simulink model "control_system"  (R2020b)
settings: Solver=FixedStepAuto  StartTime=0.0  StopTime=t_sim  FixedStep=Ts  RelTol=1e-2
values from neighbouring files (symbols this model uses):
  Hp = 10    [main_script.m]
  InitPosX = -2.4980e+03    (= -2498)    [main_script.m]
  InitPosY = -650.5503    [main_script.m]
  InitVelX = V0*cosd(InitYaw)    [main_script.m]
  InitVelY = V0*sind(InitYaw)    [main_script.m]
  InitYaw = 21    [main_script.m]
  lr = 1.592    [main_script.m]
  m = 1625    [main_script.m]
  Ts = 0.1    [main_script.m]
  V0 = 25    [main_script.m]
libraries: neural x856, simulink x1, autolibshared x1, drivingscenarioandsensors x1
(part 6 of 40)

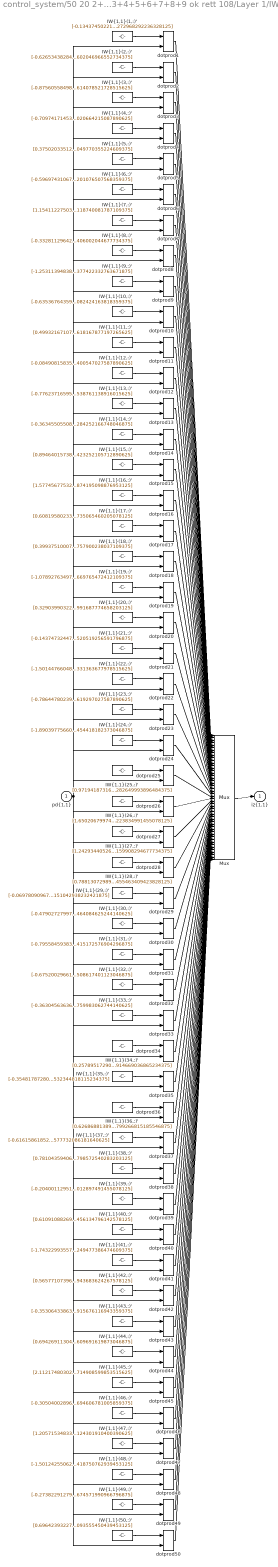
== system control_system/50 20 2+3+4+5+6+7+8+9 ok rett 108/Layer 1/IW{1,1} ==
  "pd{1,1}" : Inport  PortDimensions=9  SampleTime=0.1
      mask Display: e = 0.06;c1 = [120 230 180]/255;c2 = ([120 230 180]+0)/(256+128);c3 = ([120 230 180]+128)/(256+128);patch([0 1 1 0],[0 0 1 1],c1);patch([0 1 1 1-e 1-e 0+e],[0 0 1 1-e 0+e 0+e],c2);patch([0 0 1 1-e 0+e 0+e],[0 1 1 1-e 1-e 0+e],c3);plot([0 1 1 0 0],[0 0 1 1 0]);
  "IW{1,1}(1,:)'" : Constant  Value=[-0.1343745022107840358938091185336816124618053436279296875;-0.2201570215463205248962452742489404045045375823974609375;0.493314924472624927176411802065558731555938720703125;0.240218537769716855567736502052866853773593902587890625;0.0035729013340322856272235352292909738025628030300140380859375;1.2275952974377080106904713829862885177135467529296875;0.32609691089661685392542267436510883271694183349609375;-0.9495712296454932310751928525860421359539031982421875;-0.70107606410829692578090543975122272968292236328125]
      mask Display: e = 0.06;c1 = [120 150 230]/255;c2 = ([120 150 230]+0)/383;c3 = ([120 150 230]+128)/383;patch([0 1 1 0],[0 0 1 1],c1);patch([0 1 1 1-e 1-e 0+e],[0 0 1 1-e 0+e 0+e],c2);patch([0 0 1 1-e 0+e 0+e],[0 1 1 1-e 1-e 0+e],c3);plot([0 1 1 0 0],[0 0 1 1 0]);disp('Weights');
  "IW{1,1}(10,:)'" : Constant  Value=[-0.635367643598796494330827044905163347721099853515625;1.266134724639150999081493864650838077068328857421875;0.279110981570210359148376255689072422683238983154296875;0.6725165935042671794263924311962909996509552001953125;-0.279299335778829205256812429070123471319675445556640625;0.1298072467704776411512312961349380202591419219970703125;0.79908196252433827400096788551309145987033843994140625;1.35790638049596434910881725954823195934295654296875;0.0948926349490134268815921814166358672082424163818359375]
      mask Display: e = 0.06;c1 = [120 150 230]/255;c2 = ([120 150 230]+0)/383;c3 = ([120 150 230]+128)/383;patch([0 1 1 0],[0 0 1 1],c1);patch([0 1 1 1-e 1-e 0+e],[0 0 1 1-e 0+e 0+e],c2);patch([0 0 1 1-e 0+e 0+e],[0 1 1 1-e 1-e 0+e],c3);plot([0 1 1 0 0],[0 0 1 1 0]);disp('Weights');
  "IW{1,1}(11,:)'" : Constant  Value=[0.4993216710750658648976241238415241241455078125;0.5262356768534541817672334218514151871204376220703125;0.681666886525891246861874606111086905002593994140625;-0.87555884751066026527865915340953506529331207275390625;-0.60105755257610093966746944715850986540317535400390625;0.5843485194005146876605749639566056430339813232421875;0.96478303636410756016772438670159317553043365478515625;0.77348642815128221261744556613848544657230377197265625;-0.6497149588995887459219602533266879618167877197265625]
      mask Display: e = 0.06;c1 = [120 150 230]/255;c2 = ([120 150 230]+0)/383;c3 = ([120 150 230]+128)/383;patch([0 1 1 0],[0 0 1 1],c1);patch([0 1 1 1-e 1-e 0+e],[0 0 1 1-e 0+e 0+e],c2);patch([0 0 1 1-e 0+e 0+e],[0 1 1 1-e 1-e 0+e],c3);plot([0 1 1 0 0],[0 0 1 1 0]);disp('Weights');
  "IW{1,1}(12,:)'" : Constant  Value=[-0.084908158355977925157986874182824976742267608642578125;-0.7864413820746027905528308110660873353481292724609375;-1.011454847098846254738191419164650142192840576171875;-0.1117623118762176848139944240756449289619922637939453125;-0.207538480609310960200986073687090538442134857177734375;1.05662315566693099100348263164050877094268798828125;-1.27361323393598535602677657152526080608367919921875;-0.94238788342574653089656067095347680151462554931640625;-0.0740762271510614633829305830658995546400547027587890625]
      mask Display: e = 0.06;c1 = [120 150 230]/255;c2 = ([120 150 230]+0)/383;c3 = ([120 150 230]+128)/383;patch([0 1 1 0],[0 0 1 1],c1);patch([0 1 1 1-e 1-e 0+e],[0 0 1 1-e 0+e 0+e],c2);patch([0 0 1 1-e 0+e 0+e],[0 1 1 1-e 1-e 0+e],c3);plot([0 1 1 0 0],[0 0 1 1 0]);disp('Weights');
  "IW{1,1}(13,:)'" : Constant  Value=[-0.77623716595878800017516141451778821647167205810546875;0.01224940877890513639403291534790696459822356700897216796875;-1.1967390742769350442387121802312321960926055908203125;0.674325482748454163584028719924390316009521484375;-0.31108072366164207789296369810472242534160614013671875;-0.6359597085702881624769133850350044667720794677734375;-1.128846677766122130748271956690587103366851806640625;-0.006871567558858683588685067888945923186838626861572265625;-0.264283133847268258964646747699589468538761138916015625]
      mask Display: e = 0.06;c1 = [120 150 230]/255;c2 = ([120 150 230]+0)/383;c3 = ([120 150 230]+128)/383;patch([0 1 1 0],[0 0 1 1],c1);patch([0 1 1 1-e 1-e 0+e],[0 0 1 1-e 0+e 0+e],c2);patch([0 0 1 1-e 0+e 0+e],[0 1 1 1-e 1-e 0+e],c3);plot([0 1 1 0 0],[0 0 1 1 0]);disp('Weights');
  "IW{1,1}(14,:)'" : Constant  Value=[-0.363455055082136324617891887100995518267154693603515625;1.286478296564485201969318950432352721691131591796875;0.040608931980886768531302521978432196192443370819091796875;-0.304597316839120890730185919892392121255397796630859375;0.189441761685817888771765638011856935918331146240234375;-0.11649603633906462085700894704132224433124065399169921875;1.216577309348745306039063507341779768466949462890625;-2.649690499494823381354535740683786571025848388671875;-1.0884535716017775808239775869878940284252166748046875]
      mask Display: e = 0.06;c1 = [120 150 230]/255;c2 = ([120 150 230]+0)/383;c3 = ([120 150 230]+128)/383;patch([0 1 1 0],[0 0 1 1],c1);patch([0 1 1 1-e 1-e 0+e],[0 0 1 1-e 0+e 0+e],c2);patch([0 0 1 1-e 0+e 0+e],[0 1 1 1-e 1-e 0+e],c3);plot([0 1 1 0 0],[0 0 1 1 0]);disp('Weights');
  "IW{1,1}(15,:)'" : Constant  Value=[0.89464015738325664006680426609818823635578155517578125;0.81871186647511307032942795558483339846134185791015625;0.034969645491070143472622788749504252336919307708740234375;0.813319109544075491413650524918921291828155517578125;0.304501924088689202019253343678428791463375091552734375;1.276721925975607074832396392594091594219207763671875;0.376418920830022762924471635415102355182170867919921875;0.20670604322129293439758157546748407185077667236328125;1.1612427578136479411341497325338423252105712890625]
      mask Display: e = 0.06;c1 = [120 150 230]/255;c2 = ([120 150 230]+0)/383;c3 = ([120 150 230]+128)/383;patch([0 1 1 0],[0 0 1 1],c1);patch([0 1 1 1-e 1-e 0+e],[0 0 1 1-e 0+e 0+e],c2);patch([0 0 1 1-e 0+e 0+e],[0 1 1 1-e 1-e 0+e],c3);plot([0 1 1 0 0],[0 0 1 1 0]);disp('Weights');
  "IW{1,1}(16,:)'" : Constant  Value=[1.57745677532034367374080829904414713382720947265625;-1.1514762186593205939288964145816862583160400390625;0.9935027681728108017722433942253701388835906982421875;0.8910553917919352695520274210139177739620208740234375;0.474810013596444091543702370472601614892482757568359375;0.8601933682805522618508575760642997920513153076171875;0.332891623686451365582428252309910021722316741943359375;1.2544283751669607074319401363027282059192657470703125;-0.300158428375610075722335068348911590874195098876953125]
      mask Display: e = 0.06;c1 = [120 150 230]/255;c2 = ([120 150 230]+0)/383;c3 = ([120 150 230]+128)/383;patch([0 1 1 0],[0 0 1 1],c1);patch([0 1 1 1-e 1-e 0+e],[0 0 1 1-e 0+e 0+e],c2);patch([0 0 1 1-e 0+e 0+e],[0 1 1 1-e 1-e 0+e],c3);plot([0 1 1 0 0],[0 0 1 1 0]);disp('Weights');
  "IW{1,1}(17,:)'" : Constant  Value=[0.608195802333024726493704292806796729564666748046875;0.47127526029324162681888310544309206306934356689453125;0.36214244417380092588842899203882552683353424072265625;0.3294693882679109453448518252116627991199493408203125;-0.66612419048444915237183749923133291304111480712890625;0.5817769197731477159862834014347754418849945068359375;1.5236633537899508805679715806036256253719329833984375;-0.91766798575549302086074021644890308380126953125;0.88163371330469708642141313248430378735065460205078125]
      mask Display: e = 0.06;c1 = [120 150 230]/255;c2 = ([120 150 230]+0)/383;c3 = ([120 150 230]+128)/383;patch([0 1 1 0],[0 0 1 1],c1);patch([0 1 1 1-e 1-e 0+e],[0 0 1 1-e 0+e 0+e],c2);patch([0 0 1 1-e 0+e 0+e],[0 1 1 1-e 1-e 0+e],c3);plot([0 1 1 0 0],[0 0 1 1 0]);disp('Weights');
  "IW{1,1}(18,:)'" : Constant  Value=[0.399375100074075894962533084253664128482341766357421875;1.3435825717445688542994730596547015011310577392578125;1.5781318163517810138074537462671287357807159423828125;-0.155094863392196469220607468741945922374725341796875;1.3897167318388150558661209288402460515499114990234375;0.66382684499126110022615421257796697318553924560546875;-0.1403045882415885625693618976583820767700672149658203125;0.633292869042725303785346113727428019046783447265625;-1.19177375240624083829743540263734757900238037109375]
      mask Display: e = 0.06;c1 = [120 150 230]/255;c2 = ([120 150 230]+0)/383;c3 = ([120 150 230]+128)/383;patch([0 1 1 0],[0 0 1 1],c1);patch([0 1 1 1-e 1-e 0+e],[0 0 1 1-e 0+e 0+e],c2);patch([0 0 1 1-e 0+e 0+e],[0 1 1 1-e 1-e 0+e],c3);plot([0 1 1 0 0],[0 0 1 1 0]);disp('Weights');
  "IW{1,1}(19,:)'" : Constant  Value=[-1.0789276349723007086822690325789153575897216796875;-1.3867166392141216935129932608106173574924468994140625;0.1648811111358275127702910367588629014790058135986328125;-1.5050692494481001659778485191054642200469970703125;-0.403242892039837930173717950310674495995044708251953125;-0.0850366986317305506570818351974594406783580780029296875;0.351782679257654662396959110992611385881900787353515625;1.85432216169652708259718565386720001697540283203125;-0.399103180886815456229754772721207700669765472412109375]
      mask Display: e = 0.06;c1 = [120 150 230]/255;c2 = ([120 150 230]+0)/383;c3 = ([120 150 230]+128)/383;patch([0 1 1 0],[0 0 1 1],c1);patch([0 1 1 1-e 1-e 0+e],[0 0 1 1-e 0+e 0+e],c2);patch([0 0 1 1-e 0+e 0+e],[0 1 1 1-e 1-e 0+e],c3);plot([0 1 1 0 0],[0 0 1 1 0]);disp('Weights');
  "IW{1,1}(2,:)'" : Constant  Value=[-0.6265343828480018917304050773964263498783111572265625;-0.098149421145493020990357990740449167788028717041015625;1.9729387189784401979153471984318457543849945068359375;1.3105035919609397954133100938634015619754791259765625;-0.300689271275498715141338834655471146106719970703125;0.54673346645999842952079461610992439091205596923828125;-1.00482267753112264330184189020656049251556396484375;0.005126759769235396564657225582095634308643639087677001953125;0.402468829493407065367449604309513233602046966552734375]
      mask Display: e = 0.06;c1 = [120 150 230]/255;c2 = ([120 150 230]+0)/383;c3 = ([120 150 230]+128)/383;patch([0 1 1 0],[0 0 1 1],c1);patch([0 1 1 1-e 1-e 0+e],[0 0 1 1-e 0+e 0+e],c2);patch([0 0 1 1-e 0+e 0+e],[0 1 1 1-e 1-e 0+e],c3);plot([0 1 1 0 0],[0 0 1 1 0]);disp('Weights');
  "IW{1,1}(20,:)'" : Constant  Value=[0.32903990322955412040073497337289154529571533203125;0.58040702305057123577824995663831941783428192138671875;-1.079543369998765545147989541874267160892486572265625;0.495549709433944496339563556830398738384246826171875;0.01475849541834454471678217402086374931968748569488525390625;0.6517370707739134072511433259933255612850189208984375;0.7060091982681002686916826860397122800350189208984375;0.10264173611011488673749880717878113500773906707763671875;-1.34879506457316011847069603390991687774658203125]
      mask Display: e = 0.06;c1 = [120 150 230]/255;c2 = ([120 150 230]+0)/383;c3 = ([120 150 230]+128)/383;patch([0 1 1 0],[0 0 1 1],c1);patch([0 1 1 1-e 1-e 0+e],[0 0 1 1-e 0+e 0+e],c2);patch([0 0 1 1-e 0+e 0+e],[0 1 1 1-e 1-e 0+e],c3);plot([0 1 1 0 0],[0 0 1 1 0]);disp('Weights');
  "IW{1,1}(21,:)'" : Constant  Value=[-0.14374732447989624350981330280774272978305816650390625;-0.0402954239318593920859967738579143770039081573486328125;0.38731319765238569896581566354143433272838592529296875;1.989037631719348997449969829176552593708038330078125;0.76381127679371407790398507131612859666347503662109375;0.71549694533983487776396259505418129265308380126953125;-1.3060389462663597459624043040093965828418731689453125;-0.700024507199966450343708856962621212005615234375;-0.2408662673477610371985946358108776621520519256591796875]
      mask Display: e = 0.06;c1 = [120 150 230]/255;c2 = ([120 150 230]+0)/383;c3 = ([120 150 230]+128)/383;patch([0 1 1 0],[0 0 1 1],c1);patch([0 1 1 1-e 1-e 0+e],[0 0 1 1-e 0+e 0+e],c2);patch([0 0 1 1-e 0+e 0+e],[0 1 1 1-e 1-e 0+e],c3);plot([0 1 1 0 0],[0 0 1 1 0]);disp('Weights');
  "IW{1,1}(22,:)'" : Constant  Value=[-1.5014476604894049227567620619083754718303680419921875;-0.412754505781206815218098427067161537706851959228515625;0.76830306281267202184181996926781721413135528564453125;0.70981824529789394606638097684481181204319000244140625;-0.393729968921678608051450964921968989074230194091796875;-0.1718600999554333041974274465246708132326602935791015625;-1.9073931269723607417887478732154704630374908447265625;2.973563560321208054659791741869412362575531005859375;-0.250064300015983731473312445814372040331363677978515625]
      mask Display: e = 0.06;c1 = [120 150 230]/255;c2 = ([120 150 230]+0)/383;c3 = ([120 150 230]+128)/383;patch([0 1 1 0],[0 0 1 1],c1);patch([0 1 1 1-e 1-e 0+e],[0 0 1 1-e 0+e 0+e],c2);patch([0 0 1 1-e 0+e 0+e],[0 1 1 1-e 1-e 0+e],c3);plot([0 1 1 0 0],[0 0 1 1 0]);disp('Weights');
  "IW{1,1}(23,:)'" : Constant  Value=[-0.78644780239899658713653707309276796877384185791015625;0.2039698093212249652150802603500778786838054656982421875;-0.535590127558683182229515296057797968387603759765625;0.53857933595635765211540046948357485234737396240234375;1.3515952770876420441226173352333717048168182373046875;-2.42589564569713633801484320429153740406036376953125;-0.17670141464765565242345246588229201734066009521484375;0.044122307358018086897999410211923532187938690185546875;-1.1806380640758258326883378686034120619297027587890625]
      mask Display: e = 0.06;c1 = [120 150 230]/255;c2 = ([120 150 230]+0)/383;c3 = ([120 150 230]+128)/383;patch([0 1 1 0],[0 0 1 1],c1);patch([0 1 1 1-e 1-e 0+e],[0 0 1 1-e 0+e 0+e],c2);patch([0 0 1 1-e 0+e 0+e],[0 1 1 1-e 1-e 0+e],c3);plot([0 1 1 0 0],[0 0 1 1 0]);disp('Weights');
  "IW{1,1}(24,:)'" : Constant  Value=[-1.8903977566011811450863433492486365139484405517578125;-0.1716829364750723507793139788191183470189571380615234375;0.19568944686699929480511173096601851284503936767578125;-0.92695327627895751643194444113760255277156829833984375;-0.94439922472159576471995023894123733043670654296875;4.158514021467741628157455124892294406890869140625;-0.59169238273870117250652356233331374824047088623046875;3.865002745752950108482082214322872459888458251953125;-0.486221855689500326302976418446633033454418182373046875]
      mask Display: e = 0.06;c1 = [120 150 230]/255;c2 = ([120 150 230]+0)/383;c3 = ([120 150 230]+128)/383;patch([0 1 1 0],[0 0 1 1],c1);patch([0 1 1 1-e 1-e 0+e],[0 0 1 1-e 0+e 0+e],c2);patch([0 0 1 1-e 0+e 0+e],[0 1 1 1-e 1-e 0+e],c3);plot([0 1 1 0 0],[0 0 1 1 0]);disp('Weights');
  "IW{1,1}(25,:)'" : Constant  Value=[0.97194187316870339632401964991004206240177154541015625;0.33655565599595582693126516460324637591838836669921875;-0.732350146859455986003695215913467109203338623046875;-0.5342568270652463535697052066097967326641082763671875;0.294284086829917745919971139301196672022342681884765625;-0.380858389058827351281166784247034229338169097900390625;0.90022726195886804134715930558741092681884765625;0.388889458274653154745692518190480768680572509765625;-0.7233772643939886393127380870282649993896484375]
      mask Display: e = 0.06;c1 = [120 150 230]/255;c2 = ([120 150 230]+0)/383;c3 = ([120 150 230]+128)/383;patch([0 1 1 0],[0 0 1 1],c1);patch([0 1 1 1-e 1-e 0+e],[0 0 1 1-e 0+e 0+e],c2);patch([0 0 1 1-e 0+e 0+e],[0 1 1 1-e 1-e 0+e],c3);plot([0 1 1 0 0],[0 0 1 1 0]);disp('Weights');
  "IW{1,1}(26,:)'" : Constant  Value=[1.650206799742701679889478327822871506214141845703125;0.2751440287276978313713016177644021809101104736328125;-0.08839072554119496716307224914999096654355525970458984375;1.8091355921185316990573710427270270884037017822265625;0.88793122285300063456503494307980872690677642822265625;2.161317142218055042945934474118985235691070556640625;0.062490739860500597868675498602897278033196926116943359375;-0.728816435986441302219418503227643668651580810546875;-0.441417895919521463543588879474555142223834991455078125]
      mask Display: e = 0.06;c1 = [120 150 230]/255;c2 = ([120 150 230]+0)/383;c3 = ([120 150 230]+128)/383;patch([0 1 1 0],[0 0 1 1],c1);patch([0 1 1 1-e 1-e 0+e],[0 0 1 1-e 0+e 0+e],c2);patch([0 0 1 1-e 0+e 0+e],[0 1 1 1-e 1-e 0+e],c3);plot([0 1 1 0 0],[0 0 1 1 0]);disp('Weights');
  "IW{1,1}(27,:)'" : Constant  Value=[1.2429344052620334704073457032791338860988616943359375;0.643092034237877197000443629804067313671112060546875;-0.02543692723731975913192826510567101649940013885498046875;2.35271190603658642004347711917944252490997314453125;-0.045149049836735226370887374969242955558001995086669921875;0.51151019332570635267387615385814569890499114990234375;-0.2492781695850741774389547344981110654771327972412109375;2.47668571726079989048230345360934734344482421875;0.332171884911200032686195982023491524159908294677734375]
      mask Display: e = 0.06;c1 = [120 150 230]/255;c2 = ([120 150 230]+0)/383;c3 = ([120 150 230]+128)/383;patch([0 1 1 0],[0 0 1 1],c1);patch([0 1 1 1-e 1-e 0+e],[0 0 1 1-e 0+e 0+e],c2);patch([0 0 1 1-e 0+e 0+e],[0 1 1 1-e 1-e 0+e],c3);plot([0 1 1 0 0],[0 0 1 1 0]);disp('Weights');
  "IW{1,1}(28,:)'" : Constant  Value=[0.788130729896838300163608437287621200084686279296875;-0.2054429587058503869911874062381684780120849609375;-0.4717687480737471350522582724806852638721466064453125;-0.5514851259956536910777913362835533916950225830078125;1.2579968231444536019836277773720212280750274658203125;3.53449811365294674914139250176958739757537841796875;-0.05000756981324182282033774527008063159883022308349609375;1.066653902632202832734265030012466013431549072265625;-0.92112634419193384349711095637758262455463409423828125]
      mask Display: e = 0.06;c1 = [120 150 230]/255;c2 = ([120 150 230]+0)/383;c3 = ([120 150 230]+128)/383;patch([0 1 1 0],[0 0 1 1],c1);patch([0 1 1 1-e 1-e 0+e],[0 0 1 1-e 0+e 0+e],c2);patch([0 0 1 1-e 0+e 0+e],[0 1 1 1-e 1-e 0+e],c3);plot([0 1 1 0 0],[0 0 1 1 0]);disp('Weights');
  "IW{1,1}(29,:)'" : Constant  Value=[-0.0697809096715136245592248087632469832897186279296875;1.3531797948887407390117232353077270090579986572265625;-0.6419029163366862800188528126454912126064300537109375;-0.028841152675946106487270270690714824013411998748779296875;-0.479176304015521470347493959707207977771759033203125;-2.350572803536635557719591815839521586894989013671875;-0.80130587738460068436552319326438009738922119140625;-1.107683684106520960455100066610611975193023681640625;0.61859833911273021112009473654325120151042938232421875]
      mask Display: e = 0.06;c1 = [120 150 230]/255;c2 = ([120 150 230]+0)/383;c3 = ([120 150 230]+128)/383;patch([0 1 1 0],[0 0 1 1],c1);patch([0 1 1 1-e 1-e 0+e],[0 0 1 1-e 0+e 0+e],c2);patch([0 0 1 1-e 0+e 0+e],[0 1 1 1-e 1-e 0+e],c3);plot([0 1 1 0 0],[0 0 1 1 0]);disp('Weights');
  "IW{1,1}(3,:)'" : Constant  Value=[-0.87560558498616380962431549050961621105670928955078125;0.475208875268377572975708744706935249269008636474609375;-0.23125048510105050691976202870137058198451995849609375;0.81042970746900555578662306288606487214565277099609375;-0.00846196731237875039710605307163859833963215351104736328125;0.3162548738087338495716949182678945362567901611328125;-0.449521296222999133807007865470950491726398468017578125;-0.1640179544949538215092843529419042170047760009765625;-1.4468755556789558713859378258348442614078521728515625]
      mask Display: e = 0.06;c1 = [120 150 230]/255;c2 = ([120 150 230]+0)/383;c3 = ([120 150 230]+128)/383;patch([0 1 1 0],[0 0 1 1],c1);patch([0 1 1 1-e 1-e 0+e],[0 0 1 1-e 0+e 0+e],c2);patch([0 0 1 1-e 0+e 0+e],[0 1 1 1-e 1-e 0+e],c3);plot([0 1 1 0 0],[0 0 1 1 0]);disp('Weights');
  "IW{1,1}(30,:)'" : Constant  Value=[-0.479027279974841790899375837398110888898372650146484375;0.706989588142103553281003769370727241039276123046875;0.68721890516442041274558505392633378505706787109375;-0.208282251599368972705406122258864343166351318359375;-0.8824602696738892415595501006464473903179168701171875;1.925585047789335479961891905986703932285308837890625;2.528949615292193531246311977156437933444976806640625;1.546312974614030277820120318210683763027191162109375;0.72539840742970584930304767112829722464084625244140625]
      mask Display: e = 0.06;c1 = [120 150 230]/255;c2 = ([120 150 230]+0)/383;c3 = ([120 150 230]+128)/383;patch([0 1 1 0],[0 0 1 1],c1);patch([0 1 1 1-e 1-e 0+e],[0 0 1 1-e 0+e 0+e],c2);patch([0 0 1 1-e 0+e 0+e],[0 1 1 1-e 1-e 0+e],c3);plot([0 1 1 0 0],[0 0 1 1 0]);disp('Weights');
  "IW{1,1}(31,:)'" : Constant  Value=[-0.7955845938366306047129228318226523697376251220703125;0.302951948623523314996219824024592526257038116455078125;-0.7402939797904515284443505152012221515178680419921875;0.000853288387840656081806400834466330707073211669921875;-0.659965289742979965836866540485061705112457275390625;-3.018261355173430526832589748664759099483489990234375;-0.2471034107826629855342304153964505530893802642822265625;2.86413662430265691938302552443929016590118408203125;1.087402555219401545372193140792660415172576904296875]
      mask Display: e = 0.06;c1 = [120 150 230]/255;c2 = ([120 150 230]+0)/383;c3 = ([120 150 230]+128)/383;patch([0 1 1 0],[0 0 1 1],c1);patch([0 1 1 1-e 1-e 0+e],[0 0 1 1-e 0+e 0+e],c2);patch([0 0 1 1-e 0+e 0+e],[0 1 1 1-e 1-e 0+e],c3);plot([0 1 1 0 0],[0 0 1 1 0]);disp('Weights');
  "IW{1,1}(32,:)'" : Constant  Value=[-0.67520029661175673396655838587321341037750244140625;-0.412837749235635431688251628656871616840362548828125;-1.05785561819704110320117251831106841564178466796875;0.30923671035689392905254635479650460183620452880859375;-1.51924487732602653267122150282375514507293701171875;1.100070466424468929034219399909488856792449951171875;0.62492162787886040842266766048851422965526580810546875;-0.33030471122401772188226232174201868474483489990234375;-0.68673116558837232759060498210601508617401123046875]
      mask Display: e = 0.06;c1 = [120 150 230]/255;c2 = ([120 150 230]+0)/383;c3 = ([120 150 230]+128)/383;patch([0 1 1 0],[0 0 1 1],c1);patch([0 1 1 1-e 1-e 0+e],[0 0 1 1-e 0+e 0+e],c2);patch([0 0 1 1-e 0+e 0+e],[0 1 1 1-e 1-e 0+e],c3);plot([0 1 1 0 0],[0 0 1 1 0]);disp('Weights');
  "IW{1,1}(33,:)'" : Constant  Value=[-0.3630456363690031107438471735804341733455657958984375;-0.293172820598399941349754271868732757866382598876953125;-2.136529476080898604095636983402073383331298828125;-0.88138776302255250616468629232258535921573638916015625;1.3859742387395044271869437579880468547344207763671875;0.87569532214404788295070147796650417149066925048828125;-0.025226716696347482871143341753850108943879604339599609375;0.052432708744057705818608638992373016662895679473876953125;-0.60985735250658823503044914104975759983062744140625]
      mask Display: e = 0.06;c1 = [120 150 230]/255;c2 = ([120 150 230]+0)/383;c3 = ([120 150 230]+128)/383;patch([0 1 1 0],[0 0 1 1],c1);patch([0 1 1 1-e 1-e 0+e],[0 0 1 1-e 0+e 0+e],c2);patch([0 0 1 1-e 0+e 0+e],[0 1 1 1-e 1-e 0+e],c3);plot([0 1 1 0 0],[0 0 1 1 0]);disp('Weights');
  "IW{1,1}(34,:)'" : Constant  Value=[0.257895172904310354677903660558513365685939788818359375;-0.61990690113502300295778013605740852653980255126953125;0.531401672933585533797895550378598272800445556640625;-1.4764910132036177525804987453739158809185028076171875;-0.732921489591585650913430072250775992870330810546875;-0.98273039881687085372874435051926411688327789306640625;1.84461551588405558987915355828590691089630126953125;-5.6216731296542956641815180773846805095672607421875;-0.32490285188696910179118049200042150914669036865234375]
      mask Display: e = 0.06;c1 = [120 150 230]/255;c2 = ([120 150 230]+0)/383;c3 = ([120 150 230]+128)/383;patch([0 1 1 0],[0 0 1 1],c1);patch([0 1 1 1-e 1-e 0+e],[0 0 1 1-e 0+e 0+e],c2);patch([0 0 1 1-e 0+e 0+e],[0 1 1 1-e 1-e 0+e],c3);plot([0 1 1 0 0],[0 0 1 1 0]);disp('Weights');
  "IW{1,1}(35,:)'" : Constant  Value=[-0.35481787280470011847199884869041852653026580810546875;0.497078260792040094173671604949049651622772216796875;0.391115501772683449299705671364790759980678558349609375;0.0327190980961163668805369297842844389379024505615234375;-0.53762666975975459404679668296012096107006072998046875;-0.11201025698772511252077066501442459411919116973876953125;-1.0184435948014523010130005786777473986148834228515625;0.58936808957406683351365472844918258488178253173828125;-0.165755464487973236398232756982906721532344818115234375]
      mask Display: e = 0.06;c1 = [120 150 230]/255;c2 = ([120 150 230]+0)/383;c3 = ([120 150 230]+128)/383;patch([0 1 1 0],[0 0 1 1],c1);patch([0 1 1 1-e 1-e 0+e],[0 0 1 1-e 0+e 0+e],c2);patch([0 0 1 1-e 0+e 0+e],[0 1 1 1-e 1-e 0+e],c3);plot([0 1 1 0 0],[0 0 1 1 0]);disp('Weights');
  "IW{1,1}(36,:)'" : Constant  Value=[0.62686881389306614575929188504233025014400482177734375;1.24730954642434443968568302807398140430450439453125;-0.03217985851578696043784333369330852292478084564208984375;-0.1545692615767153277328560534442658536136150360107421875;-0.60062739392962549711540987118496559560298919677734375;-0.6083944176007214377221998802269808948040008544921875;1.25412749360978370560815164935775101184844970703125;-0.052290393032111283366791809612550423480570316314697265625;0.032940943461521536572700341594099882058799266815185546875]
      mask Display: e = 0.06;c1 = [120 150 230]/255;c2 = ([120 150 230]+0)/383;c3 = ([120 150 230]+128)/383;patch([0 1 1 0],[0 0 1 1],c1);patch([0 1 1 1-e 1-e 0+e],[0 0 1 1-e 0+e 0+e],c2);patch([0 0 1 1-e 0+e 0+e],[0 1 1 1-e 1-e 0+e],c3);plot([0 1 1 0 0],[0 0 1 1 0]);disp('Weights');
  "IW{1,1}(37,:)'" : Constant  Value=[-0.6161586185246543667659580023610033094882965087890625;-0.465772094505140066278414678890840150415897369384765625;-1.0636096376104726690670077005052007734775543212890625;-1.7097043635174504760954050652799196541309356689453125;-0.034284451933208302809585887871435261331498622894287109375;-1.5381426648641050025645427012932486832141876220703125;0.888664723820453250624495922238565981388092041015625;2.053386550122289211373072248534299433231353759765625;-0.0643003986919327419347069962896057404577732086181640625]
      mask Display: e = 0.06;c1 = [120 150 230]/255;c2 = ([120 150 230]+0)/383;c3 = ([120 150 230]+128)/383;patch([0 1 1 0],[0 0 1 1],c1);patch([0 1 1 1-e 1-e 0+e],[0 0 1 1-e 0+e 0+e],c2);patch([0 0 1 1-e 0+e 0+e],[0 1 1 1-e 1-e 0+e],c3);plot([0 1 1 0 0],[0 0 1 1 0]);disp('Weights');
  "IW{1,1}(38,:)'" : Constant  Value=[0.78104359406048884384432540173293091356754302978515625;0.040940951000542340210142100431767175905406475067138671875;-0.71202233924154534339123756581102497875690460205078125;-0.51879568600014192014668878982774913311004638671875;-1.264821397745169662130138021893799304962158203125;-0.50861084929579247759789950578124262392520904541015625;0.272379276812569681709419455728493630886077880859375;-0.0150283980679020816306756813673928263597190380096435546875;0.8847424542194499696989851145190186798572540283203125]
      mask Display: e = 0.06;c1 = [120 150 230]/255;c2 = ([120 150 230]+0)/383;c3 = ([120 150 230]+128)/383;patch([0 1 1 0],[0 0 1 1],c1);patch([0 1 1 1-e 1-e 0+e],[0 0 1 1-e 0+e 0+e],c2);patch([0 0 1 1-e 0+e 0+e],[0 1 1 1-e 1-e 0+e],c3);plot([0 1 1 0 0],[0 0 1 1 0]);disp('Weights');
  "IW{1,1}(39,:)'" : Constant  Value=[-0.204001129517059232032494264785782434046268463134765625;1.48388946688270895180039588012732565402984619140625;-0.3167231601891822290184563826187513768672943115234375;0.44364690307430365567853414177079685032367706298828125;1.4764061404163844049008957881596870720386505126953125;-1.86891152957747497254104018793441355228424072265625;0.20965317418250284386971316052949987351894378662109375;-0.6964398172337873393900053997640497982501983642578125;0.56513683668304104390500697263632901012897491455078125]
      mask Display: e = 0.06;c1 = [120 150 230]/255;c2 = ([120 150 230]+0)/383;c3 = ([120 150 230]+128)/383;patch([0 1 1 0],[0 0 1 1],c1);patch([0 1 1 1-e 1-e 0+e],[0 0 1 1-e 0+e 0+e],c2);patch([0 0 1 1-e 0+e 0+e],[0 1 1 1-e 1-e 0+e],c3);plot([0 1 1 0 0],[0 0 1 1 0]);disp('Weights');
  "IW{1,1}(4,:)'" : Constant  Value=[-0.70974171453276080345773380031459964811801910400390625;-0.7472184002806414593322870132396928966045379638671875;-1.2023833202767775230057623048196546733379364013671875;-0.1917892245454444755115019916047458536922931671142578125;0.81006788755395298107231383255566470324993133544921875;0.2385935770329483951446292167020146735012531280517578125;0.5162569777931953485250460289535112679004669189453125;0.134156673670716652946310887273284606635570526123046875;-0.887713292120228203430087887682020664215087890625]
      mask Display: e = 0.06;c1 = [120 150 230]/255;c2 = ([120 150 230]+0)/383;c3 = ([120 150 230]+128)/383;patch([0 1 1 0],[0 0 1 1],c1);patch([0 1 1 1-e 1-e 0+e],[0 0 1 1-e 0+e 0+e],c2);patch([0 0 1 1-e 0+e 0+e],[0 1 1 1-e 1-e 0+e],c3);plot([0 1 1 0 0],[0 0 1 1 0]);disp('Weights');
  "IW{1,1}(40,:)'" : Constant  Value=[0.6109108826944023018512552880565635859966278076171875;0.1134851433348192661920705859301961027085781097412109375;-0.7665821751765966585168143865303136408329010009765625;-0.67269265387908128150940001432900317013263702392578125;1.5033423418457931841629715563612990081310272216796875;3.918668443887188601593152270652353763580322265625;0.79256975088156556008556208325899206101894378662109375;0.41760567652684732475876216994947753846645355224609375;0.8162091009813174924403256227378733456134796142578125]
      mask Display: e = 0.06;c1 = [120 150 230]/255;c2 = ([120 150 230]+0)/383;c3 = ([120 150 230]+128)/383;patch([0 1 1 0],[0 0 1 1],c1);patch([0 1 1 1-e 1-e 0+e],[0 0 1 1-e 0+e 0+e],c2);patch([0 0 1 1-e 0+e 0+e],[0 1 1 1-e 1-e 0+e],c3);plot([0 1 1 0 0],[0 0 1 1 0]);disp('Weights');
  "IW{1,1}(41,:)'" : Constant  Value=[-1.743229935576636080440948717296123504638671875;-1.4311373757128456052356568761751987040042877197265625;0.6518916136115937565165268097189255058765411376953125;0.023355310903523100740653006823777104727923870086669921875;-0.0980246650668774865966526022020843811333179473876953125;-1.509270372531333226362448840518482029438018798828125;-2.422078551504594390308966467273421585559844970703125;0.09750951668167355534944107375849853269755840301513671875;1.3275731991364840833824700894183479249477386474609375]
      mask Display: e = 0.06;c1 = [120 150 230]/255;c2 = ([120 150 230]+0)/383;c3 = ([120 150 230]+128)/383;patch([0 1 1 0],[0 0 1 1],c1);patch([0 1 1 1-e 1-e 0+e],[0 0 1 1-e 0+e 0+e],c2);patch([0 0 1 1-e 0+e 0+e],[0 1 1 1-e 1-e 0+e],c3);plot([0 1 1 0 0],[0 0 1 1 0]);disp('Weights');
  "IW{1,1}(42,:)'" : Constant  Value=[0.565771073966670368093900833628140389919281005859375;-1.0093330745227906408700846441206522285938262939453125;1.49243385473924039530402296804822981357574462890625;-1.1570817881325619058685560958110727369785308837890625;-0.6398248988260319958243371729622595012187957763671875;0.61559098583450533315186703475774265825748443603515625;1.1116206127524204116951977994176559150218963623046875;-3.54958905041674910307847312651574611663818359375;0.49084347748456658155902232465450651943683624267578125]
      mask Display: e = 0.06;c1 = [120 150 230]/255;c2 = ([120 150 230]+0)/383;c3 = ([120 150 230]+128)/383;patch([0 1 1 0],[0 0 1 1],c1);patch([0 1 1 1-e 1-e 0+e],[0 0 1 1-e 0+e 0+e],c2);patch([0 0 1 1-e 0+e 0+e],[0 1 1 1-e 1-e 0+e],c3);plot([0 1 1 0 0],[0 0 1 1 0]);disp('Weights');
  "IW{1,1}(43,:)'" : Constant  Value=[-0.3530643386345151402139208585140295326709747314453125;0.56219639797748832688029096971149556338787078857421875;1.283447350617196835997901871451176702976226806640625;0.243863294661321727829772498807869851589202880859375;0.62313383657663035108953408780507743358612060546875;1.0988409561242231671229774292442016303539276123046875;0.0141977207339230616922609584662495763041079044342041015625;0.56276172689807879567780446450342424213886260986328125;-0.297748695263253038145734308272949419915676116943359375]
      mask Display: e = 0.06;c1 = [120 150 230]/255;c2 = ([120 150 230]+0)/383;c3 = ([120 150 230]+128)/383;patch([0 1 1 0],[0 0 1 1],c1);patch([0 1 1 1-e 1-e 0+e],[0 0 1 1-e 0+e 0+e],c2);patch([0 0 1 1-e 0+e 0+e],[0 1 1 1-e 1-e 0+e],c3);plot([0 1 1 0 0],[0 0 1 1 0]);disp('Weights');
  "IW{1,1}(44,:)'" : Constant  Value=[0.6942691130427716128536985706887207925319671630859375;0.2265756925917246367152557695590076036751270294189453125;1.527376164081475362621631575166247785091400146484375;-0.0276130593612169718265025863956907414831221103668212890625;-1.0785308234347308342648830148391425609588623046875;-0.7390420626780296320390561959357000887393951416015625;-0.8087526872927910392974126807530410587787628173828125;0.916833242883593246830287171178497374057769775390625;0.6302337558576478482308402817579917609691619873046875]
      mask Display: e = 0.06;c1 = [120 150 230]/255;c2 = ([120 150 230]+0)/383;c3 = ([120 150 230]+128)/383;patch([0 1 1 0],[0 0 1 1],c1);patch([0 1 1 1-e 1-e 0+e],[0 0 1 1-e 0+e 0+e],c2);patch([0 0 1 1-e 0+e 0+e],[0 1 1 1-e 1-e 0+e],c3);plot([0 1 1 0 0],[0 0 1 1 0]);disp('Weights');
  "IW{1,1}(45,:)'" : Constant  Value=[2.112174803021465319119442938244901597499847412109375;0.272656231398163917400978562000091187655925750732421875;-0.535203387873360636461939066066406667232513427734375;1.369203500411859675267578495549969375133514404296875;0.309640594882619357708364304926362819969654083251953125;-1.2789087496119544429262759877019561827182769775390625;1.047400352205652307446825943770818412303924560546875;0.89089942454226134227468492099433206021785736083984375;-0.956881177106437608159694718779064714908599853515625]
      mask Display: e = 0.06;c1 = [120 150 230]/255;c2 = ([120 150 230]+0)/383;c3 = ([120 150 230]+128)/383;patch([0 1 1 0],[0 0 1 1],c1);patch([0 1 1 1-e 1-e 0+e],[0 0 1 1-e 0+e 0+e],c2);patch([0 0 1 1-e 0+e 0+e],[0 1 1 1-e 1-e 0+e],c3);plot([0 1 1 0 0],[0 0 1 1 0]);disp('Weights');
  "IW{1,1}(46,:)'" : Constant  Value=[-0.30504002896117732301917158110882155597209930419921875;-0.40697590895609181416148203425109386444091796875;-0.948059525443387673959705352899618446826934814453125;0.256243067202603425069895592969260178506374359130859375;0.19158655560215265278856122677098028361797332763671875;1.372831884833633608877789811231195926666259765625;-1.3165481642570415754533996732789091765880584716796875;-0.1940191443094444745387505690814577974379062652587890625;0.9245017673573483474314116392633877694606781005859375]
      mask Display: e = 0.06;c1 = [120 150 230]/255;c2 = ([120 150 230]+0)/383;c3 = ([120 150 230]+128)/383;patch([0 1 1 0],[0 0 1 1],c1);patch([0 1 1 1-e 1-e 0+e],[0 0 1 1-e 0+e 0+e],c2);patch([0 0 1 1-e 0+e 0+e],[0 1 1 1-e 1-e 0+e],c3);plot([0 1 1 0 0],[0 0 1 1 0]);disp('Weights');
  "IW{1,1}(47,:)'" : Constant  Value=[1.2057153483395939286282327884691767394542694091796875;-0.93212377657996692281727746376418508589267730712890625;-1.2066653081415044113100520917214453220367431640625;-0.16671293412773457998099502219702117145061492919921875;-0.5314428473847245815164797022589482367038726806640625;0.033256524458713944414345320410575368441641330718994140625;0.32051162792968101999946384239592589437961578369140625;-0.221985681762044639864228656733757816255092620849609375;1.32134389027209753209035625332035124301910400390625]
      mask Display: e = 0.06;c1 = [120 150 230]/255;c2 = ([120 150 230]+0)/383;c3 = ([120 150 230]+128)/383;patch([0 1 1 0],[0 0 1 1],c1);patch([0 1 1 1-e 1-e 0+e],[0 0 1 1-e 0+e 0+e],c2);patch([0 0 1 1-e 0+e 0+e],[0 1 1 1-e 1-e 0+e],c3);plot([0 1 1 0 0],[0 0 1 1 0]);disp('Weights');
  "IW{1,1}(48,:)'" : Constant  Value=[-1.501242550623221205796653521247208118438720703125;1.1020300299873049265642066529835574328899383544921875;-1.455614465634394338877655172836966812610626220703125;-2.02645394117517785304016797454096376895904541015625;1.2106963579428253741099297258188016712665557861328125;-0.493105322988902250447296182755962945520877838134765625;1.2297503660993547303093009759322740137577056884765625;1.095581659184210021606986629194580018520355224609375;-0.9334065865161467190347366340574808418750762939453125]
      mask Display: e = 0.06;c1 = [120 150 230]/255;c2 = ([120 150 230]+0)/383;c3 = ([120 150 230]+128)/383;patch([0 1 1 0],[0 0 1 1],c1);patch([0 1 1 1-e 1-e 0+e],[0 0 1 1-e 0+e 0+e],c2);patch([0 0 1 1-e 0+e 0+e],[0 1 1 1-e 1-e 0+e],c3);plot([0 1 1 0 0],[0 0 1 1 0]);disp('Weights');
  "IW{1,1}(49,:)'" : Constant  Value=[-0.273822912790752492906420911822351627051830291748046875;1.7387105170071339710347047002869658172130584716796875;0.587061992641411567461773302056826651096343994140625;-1.366221274530310392236742700333707034587860107421875;0.196826890519442798677118844352662563323974609375;2.8249936900498369141132570803165435791015625;-2.2056086910325749528283267864026129245758056640625;-2.81106818254667789602763150469399988651275634765625;0.737541468895603014033213185030035674571990966796875]
      mask Display: e = 0.06;c1 = [120 150 230]/255;c2 = ([120 150 230]+0)/383;c3 = ([120 150 230]+128)/383;patch([0 1 1 0],[0 0 1 1],c1);patch([0 1 1 1-e 1-e 0+e],[0 0 1 1-e 0+e 0+e],c2);patch([0 0 1 1-e 0+e 0+e],[0 1 1 1-e 1-e 0+e],c3);plot([0 1 1 0 0],[0 0 1 1 0]);disp('Weights');
  "IW{1,1}(5,:)'" : Constant  Value=[0.375020335125967052558593195499270223081111907958984375;-0.32196765023874351907551272233831696212291717529296875;0.6551624413050858297680179020971991121768951416015625;0.1857420480424215869508230980500229634344577789306640625;0.774776965462438571563552613952197134494781494140625;1.3979887670515338538024252557079307734966278076171875;-0.511305608194094762808390441932715475559234619140625;1.0662006369119507720455430899164639413356781005859375;-0.10329268142743151803752965633975691162049770355224609375]
      mask Display: e = 0.06;c1 = [120 150 230]/255;c2 = ([120 150 230]+0)/383;c3 = ([120 150 230]+128)/383;patch([0 1 1 0],[0 0 1 1],c1);patch([0 1 1 1-e 1-e 0+e],[0 0 1 1-e 0+e 0+e],c2);patch([0 0 1 1-e 0+e 0+e],[0 1 1 1-e 1-e 0+e],c3);plot([0 1 1 0 0],[0 0 1 1 0]);disp('Weights');
  "IW{1,1}(50,:)'" : Constant  Value=[0.696423932272804524501452760887332260608673095703125;-0.7108068699398544243450714930077083408832550048828125;-1.1433229938151894256037621744326315820217132568359375;-0.0662144438543219582271603940171189606189727783203125;-0.8693715954715572902244957731454633176326751708984375;-0.11959202316048665737380218843100010417401790618896484375;-0.27553122962438647558514048796496354043483734130859375;-0.136103320695171781107291053558583371341228485107421875;0.74191818060279690616454217888531275093555450439453125]
      mask Display: e = 0.06;c1 = [120 150 230]/255;c2 = ([120 150 230]+0)/383;c3 = ([120 150 230]+128)/383;patch([0 1 1 0],[0 0 1 1],c1);patch([0 1 1 1-e 1-e 0+e],[0 0 1 1-e 0+e 0+e],c2);patch([0 0 1 1-e 0+e 0+e],[0 1 1 1-e 1-e 0+e],c3);plot([0 1 1 0 0],[0 0 1 1 0]);disp('Weights');
  "IW{1,1}(6,:)'" : Constant  Value=[-0.5969743106787934738832746006664820015430450439453125;0.61037664861964924245540942138177342712879180908203125;-0.466647656339219729648704060309682972729206085205078125;0.73630568593918244157947583516943268477916717529296875;0.2939800791317133121793858663295395672321319580078125;0.462882364823827663347088900991366244852542877197265625;1.17181131199543120402495333109982311725616455078125;1.370785468606797952162423825939185917377471923828125;-1.01263794354995351199022479704581201076507568359375]
      mask Display: e = 0.06;c1 = [120 150 230]/255;c2 = ([120 150 230]+0)/383;c3 = ([120 150 230]+128)/383;patch([0 1 1 0],[0 0 1 1],c1);patch([0 1 1 1-e 1-e 0+e],[0 0 1 1-e 0+e 0+e],c2);patch([0 0 1 1-e 0+e 0+e],[0 1 1 1-e 1-e 0+e],c3);plot([0 1 1 0 0],[0 0 1 1 0]);disp('Weights');
  "IW{1,1}(7,:)'" : Constant  Value=[1.1541122750389558593298033883911557495594024658203125;0.5287232620807547078811694518662989139556884765625;-0.120694842404742652686167048159404657781124114990234375;1.094074745299434159306883884710259735584259033203125;0.919235146736499419972687974222935736179351806640625;2.27895076551731623482055510976351797580718994140625;-0.80761216524645884629052261516335420310497283935546875;-0.330704095648042206700978340450092218816280364990234375;-0.27456811474737374823007485247217118740081787109375]
      mask Display: e = 0.06;c1 = [120 150 230]/255;c2 = ([120 150 230]+0)/383;c3 = ([120 150 230]+128)/383;patch([0 1 1 0],[0 0 1 1],c1);patch([0 1 1 1-e 1-e 0+e],[0 0 1 1-e 0+e 0+e],c2);patch([0 0 1 1-e 0+e 0+e],[0 1 1 1-e 1-e 0+e],c3);plot([0 1 1 0 0],[0 0 1 1 0]);disp('Weights');
  "IW{1,1}(8,:)'" : Constant  Value=[-0.33281129642816142943928525710362009704113006591796875;1.1793025718007819069299557668273337185382843017578125;0.49074067176078572938280331072746776044368743896484375;0.9595630213057677604382433855789713561534881591796875;0.002775338508445658429468760886038580792956054210662841796875;-0.14670677321808966997451761926640756428241729736328125;-0.1570789177527611990559108789966558106243610382080078125;0.866250040709289681473137534339912235736846923828125;0.6510933614511651423839566632523201406002044677734375]
      mask Display: e = 0.06;c1 = [120 150 230]/255;c2 = ([120 150 230]+0)/383;c3 = ([120 150 230]+128)/383;patch([0 1 1 0],[0 0 1 1],c1);patch([0 1 1 1-e 1-e 0+e],[0 0 1 1-e 0+e 0+e],c2);patch([0 0 1 1-e 0+e 0+e],[0 1 1 1-e 1-e 0+e],c3);plot([0 1 1 0 0],[0 0 1 1 0]);disp('Weights');
  "IW{1,1}(9,:)'" : Constant  Value=[-1.25311394838984124788794360938481986522674560546875;-0.62431087691206155199097338481806218624114990234375;1.4109308133277214114542630341020412743091583251953125;-2.01515145439454546050228600506670773029327392578125;-1.243430518574589083158343782997690141201019287109375;-1.207819599495781659470594604499638080596923828125;0.1829355152083460833711825443970155902206897735595703125;-0.301457500959920576821815529910963959991931915283203125;-1.820804612258143162506485168705694377422332763671875]
      mask Display: e = 0.06;c1 = [120 150 230]/255;c2 = ([120 150 230]+0)/383;c3 = ([120 150 230]+128)/383;patch([0 1 1 0],[0 0 1 1],c1);patch([0 1 1 1-e 1-e 0+e],[0 0 1 1-e 0+e 0+e],c2);patch([0 0 1 1-e 0+e 0+e],[0 1 1 1-e 1-e 0+e],c3);plot([0 1 1 0 0],[0 0 1 1 0]);disp('Weights');
  Mux : Mux  Inputs=50
      mask Display: e = 0.06;c1 = [120 150 230]/255;c2 = ([120 150 230]+0)/383;c3 = ([120 150 230]+128)/383;patch([0 1 1 0],[0 0 1 1],c1);patch([0 1 1 1-e 1-e 0+e],[0 0 1 1-e 0+e 0+e],c2);patch([0 0 1 1-e 0+e 0+e],[0 1 1 1-e 1-e 0+e],c3);plot([0 1 1 0 0],[0 0 1 1 0]);disp('Mux');
  dotprod{1..50} (50 alike) : neural/Weight Functions/dotprod
  "iz{1,1}" : Outport
      mask Display: e = 0.06;c1 = [120 230 180]/255;c2 = ([120 230 180]+0)/(256+128);c3 = ([120 230 180]+128)/(256+128);patch([0 1 1 0],[0 0 1 1],c1);patch([0 1 1 1-e 1-e 0+e],[0 0 1 1-e 0+e 0+e],c2);patch([0 0 1 1-e 0+e 0+e],[0 1 1 1-e 1-e 0+e],c3);plot([0 1 1 0 0],[0 0 1 1 0]);
  wires:
  "IW{1,1}(1,:)'"/1 -> dotprod1/1
  "pd{1,1}"/1 -> dotprod1/2, dotprod2/2, dotprod3/2, dotprod4/2, dotprod5/2, dotprod6/2, dotprod7/2, dotprod8/2, dotprod9/2, dotprod10/2, dotprod11/2, dotprod12/2, dotprod13/2, dotprod14/2, dotprod15/2, dotprod16/2, dotprod17/2, dotprod18/2, dotprod19/2, dotprod20/2, dotprod21/2, dotprod22/2, dotprod23/2, dotprod24/2, dotprod25/2, dotprod26/2, dotprod27/2, dotprod28/2, dotprod29/2, dotprod30/2, dotprod31/2, dotprod32/2, dotprod33/2, dotprod34/2, dotprod35/2, dotprod36/2, dotprod37/2, dotprod38/2, dotprod39/2, dotprod40/2, dotprod41/2, dotprod42/2, dotprod43/2, dotprod44/2, dotprod45/2, dotprod46/2, dotprod47/2, dotprod48/2, dotprod49/2, dotprod50/2
  dotprod1/1 -> Mux/1
  "IW{1,1}(2,:)'"/1 -> dotprod2/1
  dotprod2/1 -> Mux/2
  "IW{1,1}(3,:)'"/1 -> dotprod3/1
  dotprod3/1 -> Mux/3
  "IW{1,1}(4,:)'"/1 -> dotprod4/1
  dotprod4/1 -> Mux/4
  "IW{1,1}(5,:)'"/1 -> dotprod5/1
  dotprod5/1 -> Mux/5
  "IW{1,1}(6,:)'"/1 -> dotprod6/1
  dotprod6/1 -> Mux/6
  "IW{1,1}(7,:)'"/1 -> dotprod7/1
  dotprod7/1 -> Mux/7
  "IW{1,1}(8,:)'"/1 -> dotprod8/1
  dotprod8/1 -> Mux/8
  "IW{1,1}(9,:)'"/1 -> dotprod9/1
  dotprod9/1 -> Mux/9
  "IW{1,1}(10,:)'"/1 -> dotprod10/1
  dotprod10/1 -> Mux/10
  "IW{1,1}(11,:)'"/1 -> dotprod11/1
  dotprod11/1 -> Mux/11
  "IW{1,1}(12,:)'"/1 -> dotprod12/1
  dotprod12/1 -> Mux/12
  "IW{1,1}(13,:)'"/1 -> dotprod13/1
  dotprod13/1 -> Mux/13
  "IW{1,1}(14,:)'"/1 -> dotprod14/1
  dotprod14/1 -> Mux/14
  "IW{1,1}(15,:)'"/1 -> dotprod15/1
  dotprod15/1 -> Mux/15
  "IW{1,1}(16,:)'"/1 -> dotprod16/1
  dotprod16/1 -> Mux/16
  "IW{1,1}(17,:)'"/1 -> dotprod17/1
  dotprod17/1 -> Mux/17
  "IW{1,1}(18,:)'"/1 -> dotprod18/1
  dotprod18/1 -> Mux/18
  "IW{1,1}(19,:)'"/1 -> dotprod19/1
  dotprod19/1 -> Mux/19
  "IW{1,1}(20,:)'"/1 -> dotprod20/1
  dotprod20/1 -> Mux/20
  "IW{1,1}(21,:)'"/1 -> dotprod21/1
  dotprod21/1 -> Mux/21
  "IW{1,1}(22,:)'"/1 -> dotprod22/1
  dotprod22/1 -> Mux/22
  "IW{1,1}(23,:)'"/1 -> dotprod23/1
  dotprod23/1 -> Mux/23
  "IW{1,1}(24,:)'"/1 -> dotprod24/1
  dotprod24/1 -> Mux/24
  "IW{1,1}(25,:)'"/1 -> dotprod25/1
  dotprod25/1 -> Mux/25
  "IW{1,1}(26,:)'"/1 -> dotprod26/1
  dotprod26/1 -> Mux/26
  "IW{1,1}(27,:)'"/1 -> dotprod27/1
  dotprod27/1 -> Mux/27
  "IW{1,1}(28,:)'"/1 -> dotprod28/1
  dotprod28/1 -> Mux/28
  "IW{1,1}(29,:)'"/1 -> dotprod29/1
  dotprod29/1 -> Mux/29
  "IW{1,1}(30,:)'"/1 -> dotprod30/1
  dotprod30/1 -> Mux/30
  "IW{1,1}(31,:)'"/1 -> dotprod31/1
  dotprod31/1 -> Mux/31
  "IW{1,1}(32,:)'"/1 -> dotprod32/1
  dotprod32/1 -> Mux/32
  "IW{1,1}(33,:)'"/1 -> dotprod33/1
  dotprod33/1 -> Mux/33
  "IW{1,1}(34,:)'"/1 -> dotprod34/1
  dotprod34/1 -> Mux/34
  "IW{1,1}(35,:)'"/1 -> dotprod35/1
  dotprod35/1 -> Mux/35
  "IW{1,1}(36,:)'"/1 -> dotprod36/1
  dotprod36/1 -> Mux/36
  "IW{1,1}(37,:)'"/1 -> dotprod37/1
  dotprod37/1 -> Mux/37
  "IW{1,1}(38,:)'"/1 -> dotprod38/1
  dotprod38/1 -> Mux/38
  "IW{1,1}(39,:)'"/1 -> dotprod39/1
  dotprod39/1 -> Mux/39
  "IW{1,1}(40,:)'"/1 -> dotprod40/1
  dotprod40/1 -> Mux/40
  "IW{1,1}(41,:)'"/1 -> dotprod41/1
  dotprod41/1 -> Mux/41
  "IW{1,1}(42,:)'"/1 -> dotprod42/1
  dotprod42/1 -> Mux/42
  "IW{1,1}(43,:)'"/1 -> dotprod43/1
  dotprod43/1 -> Mux/43
  "IW{1,1}(44,:)'"/1 -> dotprod44/1
  dotprod44/1 -> Mux/44
  "IW{1,1}(45,:)'"/1 -> dotprod45/1
  dotprod45/1 -> Mux/45
  "IW{1,1}(46,:)'"/1 -> dotprod46/1
  dotprod46/1 -> Mux/46
  "IW{1,1}(47,:)'"/1 -> dotprod47/1
  dotprod47/1 -> Mux/47
  "IW{1,1}(48,:)'"/1 -> dotprod48/1
  dotprod48/1 -> Mux/48
  "IW{1,1}(49,:)'"/1 -> dotprod49/1
  dotprod49/1 -> Mux/49
  "IW{1,1}(50,:)'"/1 -> dotprod50/1
  dotprod50/1 -> Mux/50
  Mux/1 -> "iz{1,1}"/1

== system control_system/50 20 2+3+4+5+6+7+8+9 ok rett 108/Layer 2/Delays 1 ==
  "p{2}" : Inport  PortDimensions=50  SampleTime=0.1
      mask Display: e = 0.06;c1 = [120 230 180]/255;c2 = ([120 230 180]+0)/(256+128);c3 = ([120 230 180]+128)/(256+128);patch([0 1 1 0],[0 0 1 1],c1);patch([0 1 1 1-e 1-e 0+e],[0 0 1 1-e 0+e 0+e],c2);patch([0 0 1 1-e 0+e 0+e],[0 1 1 1-e 1-e 0+e],c3);plot([0 1 1 0 0],[0 0 1 1 0]);
  mux : Mux  Inputs=1
      mask Display: e = 0.06;c1 = [120 150 230]/255;c2 = ([120 150 230]+0)/383;c3 = ([120 150 230]+128)/383;patch([0 1 1 0],[0 0 1 1],c1);patch([0 1 1 1-e 1-e 0+e],[0 0 1 1-e 0+e 0+e],c2);patch([0 0 1 1-e 0+e 0+e],[0 1 1 1-e 1-e 0+e],c3);plot([0 1 1 0 0],[0 0 1 1 0]);disp('Mux')
  "pd{2,1}" : Outport
      mask Display: e = 0.06;c1 = [120 230 180]/255;c2 = ([120 230 180]+0)/(256+128);c3 = ([120 230 180]+128)/(256+128);patch([0 1 1 0],[0 0 1 1],c1);patch([0 1 1 1-e 1-e 0+e],[0 0 1 1-e 0+e 0+e],c2);patch([0 0 1 1-e 0+e 0+e],[0 1 1 1-e 1-e 0+e],c3);plot([0 1 1 0 0],[0 0 1 1 0]);
  wires:
  "p{2}"/1 -> mux/1
  mux/1 -> "pd{2,1}"/1
